simulink subsystem "Circuit_ROM_InputNoise"  (R2022a)
settings: Solver=VariableStepAuto  StartTime=0.0  StopTime=10.0  RelTol=1e-3
values from neighbouring files (symbols this model uses):
  A_ROM = est_sys.A    [RunSimulink.m]
  B_ROM = est_sys.B    [RunSimulink.m]
  C_des_ROM = est_sys.C    [RunSimulink.m]
  C_m_ROM = C_des_ROM    [RunSimulink.m]
  x_0_ROM = C_des_ROM\y_0    [RunSimulink.m]
undefined symbols (not defined in the file or in its folder): tc, Ts
libraries: simulink x2
settings Model: Creator=tyevans  LastModifiedBy=tyevans

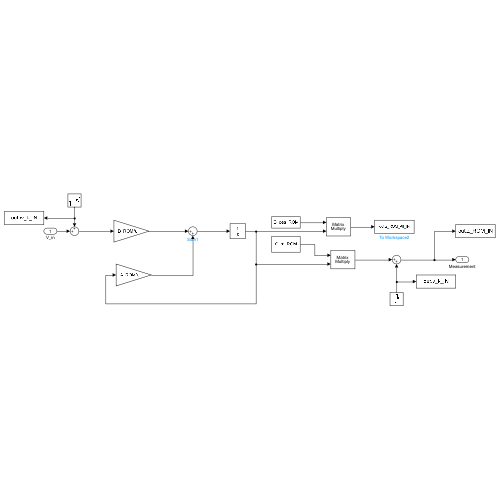
[thumbnail: Simulink's stored preview of the top-level diagram]
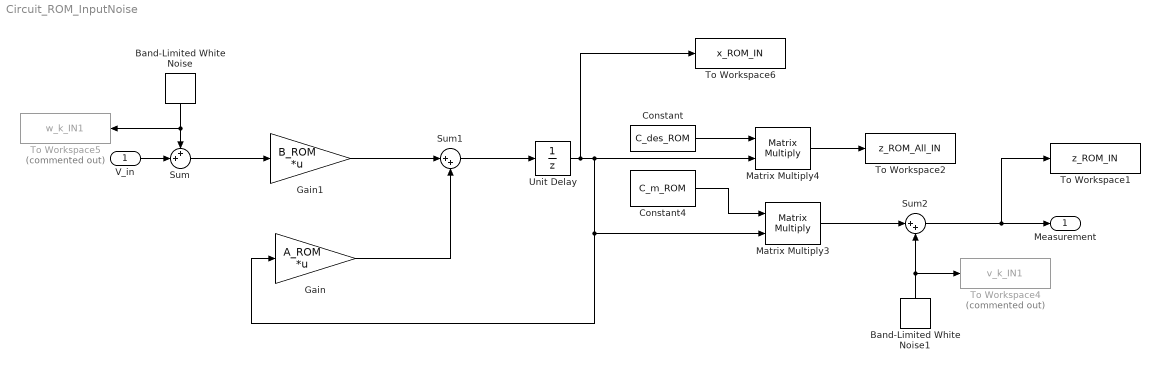
== system Circuit_ROM_InputNoise ==
  V_in : Inport
  Band-Limited White Noise : simulink/Sources/Band-Limited White Noise  Cov=pow_Q3i  Ts=tc  seed=[1]  VectorParams1D=off
  Band-Limited White Noise1 : simulink/Sources/Band-Limited White Noise  Cov=pow_R  Ts=tc  seed=[23341]  VectorParams1D=off
  Constant : Constant  Value=C_des_ROM  VectorParams1D=off
  Constant4 : Constant  Value=C_m_ROM  VectorParams1D=off
  Gain : Gain  Gain=A_ROM  Multiplication=Matrix(K*u)
  Gain1 : Gain  Gain=B_ROM  Multiplication=Matrix(K*u)
  Matrix Multiply3 : Product  Multiplication=Matrix(*)
  Matrix Multiply4 : Product  Multiplication=Matrix(*)
  Sum : Sum  Inputs=++|
  Sum1 : Sum  Inputs=|++
  Sum2 : Sum  Inputs=|++
  To Workspace1 : ToWorkspace  VariableName=z_ROM_IN  SaveFormat=Structure With Time  SampleTime=Ts
  To Workspace2 : ToWorkspace  VariableName=z_ROM_All_IN  SaveFormat=Structure With Time  SampleTime=Ts
  To Workspace4 : ToWorkspace  Commented=on  VariableName=v_k_IN1  SaveFormat=Structure With Time  SampleTime=-1
  To Workspace5 : ToWorkspace  Commented=on  VariableName=w_k_IN1  SaveFormat=Structure With Time  SampleTime=-1
      settings: Save2DSignal=2-D array (concatenate along first dimension)
  To Workspace6 : ToWorkspace  VariableName=x_ROM_IN  SaveFormat=Structure With Time  SampleTime=Ts
  Unit Delay : UnitDelay  InitialCondition=x_0_ROM  SampleTime=-1  HasFrameUpgradeWarning=on
  Measurement : Outport
  wires:
  Sum/1 -> Gain1/1
  V_in/1 -> Sum/2
  Band-Limited White Noise/1 -> Sum/1, To Workspace5/1
  Gain1/1 -> Sum1/1
  Gain/1 -> Sum1/2
  Sum1/1 -> Unit Delay/1
  Matrix Multiply4/1 -> To Workspace2/1
  Constant/1 -> Matrix Multiply4/1
  Matrix Multiply3/1 -> Sum2/1
  Constant4/1 -> Matrix Multiply3/1
  Band-Limited White Noise1/1 -> Sum2/2, To Workspace4/1
  Sum2/1 -> To Workspace1/1, Measurement/1
  Unit Delay/1 -> Gain/1, Matrix Multiply3/2, Matrix Multiply4/2, To Workspace6/1
